simulink model "Leader"  (R2024b)
settings: Solver=ode4  StartTime=0  StopTime=100  FixedStep=0.001  RelTol=1e-3
undefined symbols (not defined in the file or in its folder): DiscIntNeverNeededParam
libraries: simulink x22, vrlib x1
(part 2 of 4)

== system Leader/Ardupilot Attitude Controller/Rate Controller/PID Pitch Rate/RAT_FLTT ==
  note: See AP_Math.cpp, calc_lowpass_alpha_dt()
  note: See AC_PID.cpp, update_all()
  note: Digital Filter:
      | $y_n = (1 - \alpha)y_{n-1} + x \cdot \alpha$
  note: Alpha Calculation: (Eqn is wrong, implementation is correct)
      | $\alpha = \frac{\mathrm{d}t}{\mathrm{d}t + 2 \pi T_{\mathrm{Cutoff}}$
  u : Inport
  cutoff_freq : Inport  Port=2
  ATC Sampling Time : Constant  Value=0.01
  Add : Sum
  Calculate Alpha : Product  Inputs=*/
  Compare To Zero : simulink/Logic and Bit Operations/Compare To Zero  relop=<=  OutDataTypeStr=boolean
  Compare To Zero1 : simulink/Logic and Bit Operations/Compare To Zero  relop=<=  OutDataTypeStr=boolean
  Constant2 : Constant
  Constant3 : Constant
  Constant4 : Constant
  Divide : Product  Inputs=*/
  Gain : Gain  Gain=2*pi
  Logical Operator : Logic  Operator=OR  AllPortsSameDT=off  OutDataTypeStr=boolean
  Product : Product
  Product1 : Product
  Subtract1 : Sum  Inputs=+-
  Sum : Sum  Inputs=++|  OutDataTypeStr=double
  Switch : Switch  Criteria=u2 > Threshold  SaturateOnIntegerOverflow=off  InputSameDT=off
  Unit Delay : UnitDelay  SampleTime=-1  HasFrameUpgradeWarning=on
  y : Outport
  wires:
  Constant4/1 -> Switch/1
  Logical Operator/1 -> Switch/2
  Compare To Zero1/1 -> Logical Operator/2
  Compare To Zero/1 -> Logical Operator/1
  [cutoff_freq] -> Compare To Zero1/1
  [dt] -> Compare To Zero/1
  Switch/1 -> [alpha]
  Product/1 -> Sum/1
  u/1 -> Product/2
  cutoff_freq/1 -> [cutoff_freq]
  [dt] -> Calculate Alpha/1, Add/1
  Add/1 -> Calculate Alpha/2
  Calculate Alpha/1 -> Switch/3
  [alpha] -> Product/1
  Constant2/1 -> Subtract1/1
  [alpha] -> Subtract1/2
  Subtract1/1 -> Product1/1
  Product1/1 -> Sum/2
  Unit Delay/1 -> Product1/2
  Sum/1 -> y/1, Unit Delay/1
  ATC Sampling Time/1 -> [dt]
  Constant3/1 -> Divide/1
  [cutoff_freq] -> Gain/1
  Gain/1 -> Divide/2
  Divide/1 -> Add/2

== system Leader/Ardupilot Attitude Controller/Rate Controller/PID Roll Rate/Calc Derivative ==
  e : Inport
  ATC Sampling Time : Constant  Value=0.01
  Divide : Product  Inputs=*/
  Sum : Sum  Inputs=|+-  OutDataTypeStr=double
  Unit Delay : UnitDelay  SampleTime=-1  HasFrameUpgradeWarning=on
  derivative : Outport
  wires:
  e/1 -> Sum/1, Unit Delay/1
  Unit Delay/1 -> Sum/2
  Sum/1 -> Divide/1
  Divide/1 -> derivative/1
  ATC Sampling Time/1 -> Divide/2

== system Leader/Ardupilot Attitude Controller/Rate Controller/PID Roll Rate/I ==
  note: Integrator, see AC_PID::update_i()
  e : Inport
  limitFlg : Inport  Port=2
  ki : Inport  Port=3
  i_max : Inport  Port=4
  ATC Sampling Time : Constant  Value=0.01
  Cast To Double : DataTypeConversion  OutDataTypeStr=double  SaturateOnIntegerOverflow=off  RndMeth=Floor
  Integrator : MATLAB Function  TreatAsAtomicUnit=on
  Unit Delay1 : UnitDelay  InitialCondition=0.0  SampleTime=-1  HasFrameUpgradeWarning=on
  integrator : Outport
  wires:
  [integrator_out] -> integrator/1
  ki/1 -> Integrator/4(ki)
  i_max/1 -> Integrator/5(i_max)
  e/1 -> Integrator/1(error)
  ATC Sampling Time/1 -> Integrator/6(dt)
  limitFlg/1 -> Integrator/3(limit_flg)
  [integrator_out] -> Unit Delay1/1
  Unit Delay1/1 -> Integrator/2(integrator)
  Integrator/1(integrator_out) -> Cast To Double/1
  Cast To Double/1 -> [integrator_out]

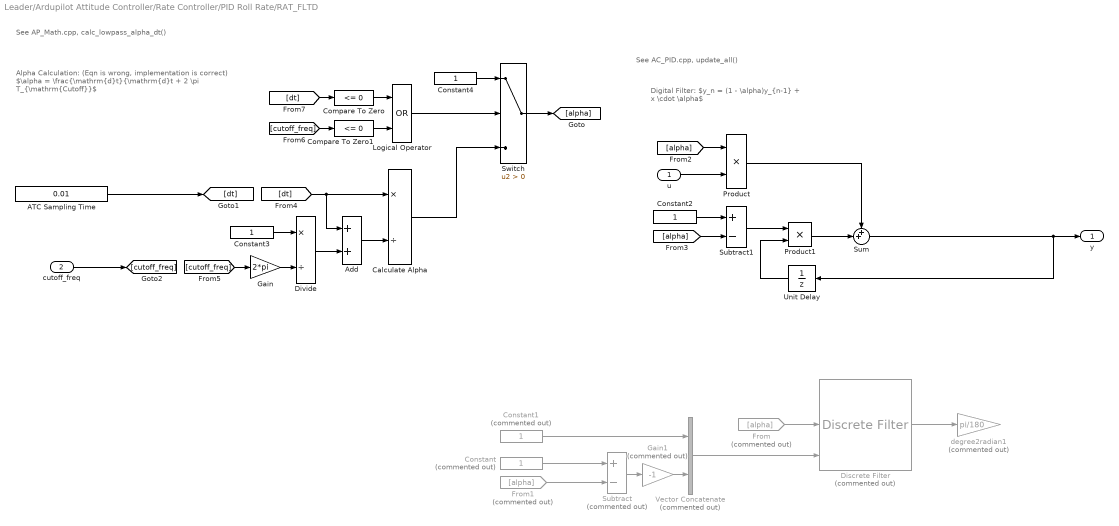
== system Leader/Ardupilot Attitude Controller/Rate Controller/PID Roll Rate/RAT_FLTD ==
  note: Digital Filter:
      | $y_n = (1 - \alpha)y_{n-1} + x \cdot \alpha$
  note: See AC_PID.cpp, update_all()
  note: See AP_Math.cpp, calc_lowpass_alpha_dt()
  note: Alpha Calculation: (Eqn is wrong, implementation is correct)
      | $\alpha = \frac{\mathrm{d}t}{\mathrm{d}t + 2 \pi T_{\mathrm{Cutoff}}$
  u : Inport
  cutoff_freq : Inport  Port=2
  ATC Sampling Time : Constant  Value=0.01
  Add : Sum
  Calculate Alpha : Product  Inputs=*/
  Compare To Zero : simulink/Logic and Bit Operations/Compare To Zero  relop=<=  OutDataTypeStr=boolean
  Compare To Zero1 : simulink/Logic and Bit Operations/Compare To Zero  relop=<=  OutDataTypeStr=boolean
  Constant : Constant  Commented=on
  Constant1 : Constant  Commented=on
  Constant2 : Constant
  Constant3 : Constant
  Constant4 : Constant
  Discrete Filter : DiscreteFilter  Commented=on  NumeratorSource=Input port  DenominatorSource=Input port  a0EqualsOne=on
      settings: InputPortMap=u0,p1,p3
  Divide : Product  Inputs=*/
  From : From  Commented=on  GotoTag=alpha
  From1 : From  Commented=on  GotoTag=alpha
  Gain : Gain  Gain=2*pi
  Gain1 : Gain  Commented=on  Gain=-1
  Logical Operator : Logic  Operator=OR  AllPortsSameDT=off  OutDataTypeStr=boolean
  Product : Product
  Product1 : Product
  Subtract : Sum  Commented=on  Inputs=+-
  Subtract1 : Sum  Inputs=+-
  Sum : Sum  Inputs=++|  OutDataTypeStr=double  AccumDataTypeStr=double
  Switch : Switch  Criteria=u2 > Threshold  SaturateOnIntegerOverflow=off  InputSameDT=off
  Unit Delay : UnitDelay  SampleTime=-1  HasFrameUpgradeWarning=on
  Vector Concatenate : Concatenate  Commented=on
  degree2radian1 : Gain  Commented=on  Gain=pi/180
  y : Outport
  wires:
  Product1/1 -> Sum/2
  Unit Delay/1 -> Product1/2
  Subtract1/1 -> Product1/1
  [alpha] -> Subtract1/2
  Constant2/1 -> Subtract1/1
  [alpha] -> Product/1
  Vector Concatenate/1 -> Discrete Filter/3
  Constant1/1 -> Vector Concatenate/1
  Gain1/1 -> Vector Concatenate/2
  Subtract/1 -> Gain1/1
  Constant/1 -> Subtract/1
  From1/1 -> Subtract/2
  From/1 -> Discrete Filter/2
  Calculate Alpha/1 -> Switch/3
  Add/1 -> Calculate Alpha/2
  [dt] -> Add/1, Calculate Alpha/1
  Gain/1 -> Divide/2
  cutoff_freq/1 -> [cutoff_freq]
  Discrete Filter/1 -> degree2radian1/1
  u/1 -> Product/2
  Divide/1 -> Add/2
  Constant3/1 -> Divide/1
  Product/1 -> Sum/1
  Switch/1 -> [alpha]
  [cutoff_freq] -> Gain/1
  [dt] -> Compare To Zero/1
  [cutoff_freq] -> Compare To Zero1/1
  Compare To Zero/1 -> Logical Operator/1
  Compare To Zero1/1 -> Logical Operator/2
  Logical Operator/1 -> Switch/2
  Constant4/1 -> Switch/1
  Sum/1 -> Unit Delay/1, y/1
  ATC Sampling Time/1 -> [dt]

== system Leader/Ardupilot Attitude Controller/Rate Controller/PID Roll Rate/RAT_FLTE ==
  note: Digital Filter:
      | $y_n = (1 - \alpha)y_{n-1} + x \cdot \alpha$
  note: See AC_PID.cpp, update_all()
  note: See AP_Math.cpp, calc_lowpass_alpha_dt()
  note: Alpha Calculation: (Eqn is wrong, implementation is correct)
      | $\alpha = \frac{\mathrm{d}t}{\mathrm{d}t + 2 \pi T_{\mathrm{Cutoff}}$
  u : Inport
  cutoff_freq : Inport  Port=2
  ATC Sampling Time : Constant  Value=0.01
  Add : Sum
  Calculate Alpha : Product  Inputs=*/
  Compare To Zero : simulink/Logic and Bit Operations/Compare To Zero  relop=<=  OutDataTypeStr=boolean
  Compare To Zero1 : simulink/Logic and Bit Operations/Compare To Zero  relop=<=  OutDataTypeStr=boolean
  Constant2 : Constant
  Constant3 : Constant
  Constant4 : Constant
  Divide : Product  Inputs=*/
  Gain : Gain  Gain=2*pi
  Logical Operator : Logic  Operator=OR  AllPortsSameDT=off  OutDataTypeStr=boolean
  Product : Product
  Product1 : Product
  Subtract1 : Sum  Inputs=+-
  Sum : Sum  Inputs=++|  OutDataTypeStr=double
  Switch : Switch  Criteria=u2 > Threshold  SaturateOnIntegerOverflow=off  InputSameDT=off
  Unit Delay : UnitDelay  SampleTime=-1  HasFrameUpgradeWarning=on
  y : Outport
  wires:
  Product1/1 -> Sum/2
  Unit Delay/1 -> Product1/2
  Subtract1/1 -> Product1/1
  [alpha] -> Subtract1/2
  Constant2/1 -> Subtract1/1
  [alpha] -> Product/1
  Calculate Alpha/1 -> Switch/3
  Add/1 -> Calculate Alpha/2
  [dt] -> Add/1, Calculate Alpha/1
  cutoff_freq/1 -> [cutoff_freq]
  u/1 -> Product/2
  Product/1 -> Sum/1
  Switch/1 -> [alpha]
  [dt] -> Compare To Zero/1
  [cutoff_freq] -> Compare To Zero1/1
  Compare To Zero/1 -> Logical Operator/1
  Compare To Zero1/1 -> Logical Operator/2
  Logical Operator/1 -> Switch/2
  Constant4/1 -> Switch/1
  Sum/1 -> Unit Delay/1, y/1
  ATC Sampling Time/1 -> [dt]
  [cutoff_freq] -> Gain/1
  Divide/1 -> Add/2
  Constant3/1 -> Divide/1
  Gain/1 -> Divide/2

== system Leader/Ardupilot Attitude Controller/Rate Controller/PID Roll Rate/RAT_FLTT ==
  note: See AP_Math.cpp, calc_lowpass_alpha_dt()
  note: See AC_PID.cpp, update_all()
  note: Digital Filter:
      | $y_n = (1 - \alpha)y_{n-1} + x \cdot \alpha$
  note: Alpha Calculation: (Eqn is wrong, implementation is correct)
      | $\alpha = \frac{\mathrm{d}t}{\mathrm{d}t + 2 \pi T_{\mathrm{Cutoff}}$
  u : Inport
  cutoff_freq : Inport  Port=2
  ATC Sampling Time : Constant  Value=0.01
  Add : Sum
  Calculate Alpha : Product  Inputs=*/
  Compare To Zero : simulink/Logic and Bit Operations/Compare To Zero  relop=<=  OutDataTypeStr=boolean
  Compare To Zero1 : simulink/Logic and Bit Operations/Compare To Zero  relop=<=  OutDataTypeStr=boolean
  Constant2 : Constant
  Constant3 : Constant
  Constant4 : Constant
  Divide : Product  Inputs=*/
  Gain : Gain  Gain=2*pi
  Logical Operator : Logic  Operator=OR  AllPortsSameDT=off  OutDataTypeStr=boolean
  Product : Product
  Product1 : Product
  Subtract1 : Sum  Inputs=+-
  Sum : Sum  Inputs=++|  OutDataTypeStr=double
  Switch : Switch  Criteria=u2 > Threshold  SaturateOnIntegerOverflow=off  InputSameDT=off
  Unit Delay : UnitDelay  SampleTime=-1  HasFrameUpgradeWarning=on
  y : Outport
  wires:
  Constant4/1 -> Switch/1
  Logical Operator/1 -> Switch/2
  Compare To Zero1/1 -> Logical Operator/2
  Compare To Zero/1 -> Logical Operator/1
  [cutoff_freq] -> Compare To Zero1/1
  [dt] -> Compare To Zero/1
  Switch/1 -> [alpha]
  Product/1 -> Sum/1
  u/1 -> Product/2
  cutoff_freq/1 -> [cutoff_freq]
  [dt] -> Calculate Alpha/1, Add/1
  Add/1 -> Calculate Alpha/2
  Calculate Alpha/1 -> Switch/3
  [alpha] -> Product/1
  Constant2/1 -> Subtract1/1
  [alpha] -> Subtract1/2
  Subtract1/1 -> Product1/1
  Product1/1 -> Sum/2
  Unit Delay/1 -> Product1/2
  Sum/1 -> y/1, Unit Delay/1
  ATC Sampling Time/1 -> [dt]
  Constant3/1 -> Divide/1
  [cutoff_freq] -> Gain/1
  Gain/1 -> Divide/2
  Divide/1 -> Add/2

== system Leader/Ardupilot Attitude Controller/Rate Controller/PID Yaw Rate/Calc Derivative ==
  e : Inport
  ATC Sampling Time : Constant  Value=0.01
  Divide : Product  Inputs=*/
  Sum : Sum  Inputs=|+-  OutDataTypeStr=double
  Unit Delay : UnitDelay  SampleTime=-1  HasFrameUpgradeWarning=on
  derivative : Outport
  wires:
  e/1 -> Sum/1, Unit Delay/1
  Unit Delay/1 -> Sum/2
  Sum/1 -> Divide/1
  Divide/1 -> derivative/1
  ATC Sampling Time/1 -> Divide/2

== system Leader/Ardupilot Attitude Controller/Rate Controller/PID Yaw Rate/I ==
  note: Integrator, see AC_PID::update_i()
  e : Inport
  limitFlg : Inport  Port=2
  ki : Inport  Port=3
  i_max : Inport  Port=4
  ATC Sampling Time : Constant  Value=0.01
  Integrator : MATLAB Function  TreatAsAtomicUnit=on
  Unit Delay1 : UnitDelay  SampleTime=-1  HasFrameUpgradeWarning=on
  integrator : Outport
  wires:
  [integrator_out] -> integrator/1
  [integrator_out] -> Unit Delay1/1
  Integrator/1(integrator_out) -> [integrator_out]
  Unit Delay1/1 -> Integrator/2(integrator)
  ki/1 -> Integrator/4(ki)
  i_max/1 -> Integrator/5(i_max)
  e/1 -> Integrator/1(error)
  ATC Sampling Time/1 -> Integrator/6(dt)
  limitFlg/1 -> Integrator/3(limit_flg)

== system Leader/Ardupilot Attitude Controller/Rate Controller/PID Yaw Rate/RAT_FLTD ==
  note: Digital Filter:
      | $y_n = (1 - \alpha)y_{n-1} + x \cdot \alpha$
  note: See AC_PID.cpp, update_all()
  note: See AP_Math.cpp, calc_lowpass_alpha_dt()
  note: Alpha Calculation: (Eqn is wrong, implementation is correct)
      | $\alpha = \frac{\mathrm{d}t}{\mathrm{d}t + 2 \pi T_{\mathrm{Cutoff}}$
  u : Inport
  cutoff_freq : Inport  Port=2
  ATC Sampling Time : Constant  Value=0.01
  Add : Sum
  Calculate Alpha : Product  Inputs=*/
  Compare To Zero : simulink/Logic and Bit Operations/Compare To Zero  relop=<=  OutDataTypeStr=boolean
  Compare To Zero1 : simulink/Logic and Bit Operations/Compare To Zero  relop=<=  OutDataTypeStr=boolean
  Constant2 : Constant
  Constant3 : Constant
  Constant4 : Constant
  Divide : Product  Inputs=*/
  Gain : Gain  Gain=2*pi
  Logical Operator : Logic  Operator=OR  AllPortsSameDT=off  OutDataTypeStr=boolean
  Product : Product
  Product1 : Product
  Subtract1 : Sum  Inputs=+-
  Sum : Sum  Inputs=++|  OutDataTypeStr=double
  Switch : Switch  Criteria=u2 > Threshold  SaturateOnIntegerOverflow=off  InputSameDT=off
  Unit Delay : UnitDelay  SampleTime=-1  HasFrameUpgradeWarning=on
  y : Outport
  wires:
  Product1/1 -> Sum/2
  Unit Delay/1 -> Product1/2
  Subtract1/1 -> Product1/1
  [alpha] -> Subtract1/2
  Constant2/1 -> Subtract1/1
  [alpha] -> Product/1
  Calculate Alpha/1 -> Switch/3
  Add/1 -> Calculate Alpha/2
  [dt] -> Add/1, Calculate Alpha/1
  Gain/1 -> Divide/2
  cutoff_freq/1 -> [cutoff_freq]
  u/1 -> Product/2
  Divide/1 -> Add/2
  Constant3/1 -> Divide/1
  Product/1 -> Sum/1
  Switch/1 -> [alpha]
  [cutoff_freq] -> Gain/1
  [dt] -> Compare To Zero/1
  [cutoff_freq] -> Compare To Zero1/1
  Compare To Zero/1 -> Logical Operator/1
  Compare To Zero1/1 -> Logical Operator/2
  Logical Operator/1 -> Switch/2
  Constant4/1 -> Switch/1
  Sum/1 -> Unit Delay/1, y/1
  ATC Sampling Time/1 -> [dt]

== system Leader/Ardupilot Attitude Controller/Rate Controller/PID Yaw Rate/RAT_FLTE ==
  note: Digital Filter:
      | $y_n = (1 - \alpha)y_{n-1} + x \cdot \alpha$
  note: See AC_PID.cpp, update_all()
  note: See AP_Math.cpp, calc_lowpass_alpha_dt()
  note: Alpha Calculation: (Eqn is wrong, implementation is correct)
      | $\alpha = \frac{\mathrm{d}t}{\mathrm{d}t + 2 \pi T_{\mathrm{Cutoff}}$
  u : Inport
  cutoff_freq : Inport  Port=2
  ATC Sampling Time : Constant  Value=0.01
  Add : Sum
  Calculate Alpha : Product  Inputs=*/
  Compare To Zero : simulink/Logic and Bit Operations/Compare To Zero  relop=<=  OutDataTypeStr=boolean
  Compare To Zero1 : simulink/Logic and Bit Operations/Compare To Zero  relop=<=  OutDataTypeStr=boolean
  Constant2 : Constant
  Constant3 : Constant
  Constant4 : Constant
  Divide : Product  Inputs=*/
  Gain : Gain  Gain=2*pi
  Logical Operator : Logic  Operator=OR  AllPortsSameDT=off  OutDataTypeStr=boolean
  Product : Product
  Product1 : Product
  Subtract1 : Sum  Inputs=+-
  Sum : Sum  Inputs=++|  OutDataTypeStr=double
  Switch : Switch  Criteria=u2 > Threshold  SaturateOnIntegerOverflow=off  InputSameDT=off
  Unit Delay : UnitDelay  SampleTime=-1  HasFrameUpgradeWarning=on
  y : Outport
  wires:
  Product1/1 -> Sum/2
  Unit Delay/1 -> Product1/2
  Subtract1/1 -> Product1/1
  [alpha] -> Subtract1/2
  Constant2/1 -> Subtract1/1
  [alpha] -> Product/1
  Calculate Alpha/1 -> Switch/3
  Add/1 -> Calculate Alpha/2
  [dt] -> Add/1, Calculate Alpha/1
  cutoff_freq/1 -> [cutoff_freq]
  u/1 -> Product/2
  Product/1 -> Sum/1
  Switch/1 -> [alpha]
  [dt] -> Compare To Zero/1
  [cutoff_freq] -> Compare To Zero1/1
  Compare To Zero/1 -> Logical Operator/1
  Compare To Zero1/1 -> Logical Operator/2
  Logical Operator/1 -> Switch/2
  Constant4/1 -> Switch/1
  Sum/1 -> Unit Delay/1, y/1
  ATC Sampling Time/1 -> [dt]
  [cutoff_freq] -> Gain/1
  Divide/1 -> Add/2
  Constant3/1 -> Divide/1
  Gain/1 -> Divide/2

== system Leader/Ardupilot Attitude Controller/Rate Controller/PID Yaw Rate/RAT_FLTT ==
  note: See AP_Math.cpp, calc_lowpass_alpha_dt()
  note: See AC_PID.cpp, update_all()
  note: Digital Filter:
      | $y_n = (1 - \alpha)y_{n-1} + x \cdot \alpha$
  note: Alpha Calculation: (Eqn is wrong, implementation is correct)
      | $\alpha = \frac{\mathrm{d}t}{\mathrm{d}t + 2 \pi T_{\mathrm{Cutoff}}$
  u : Inport
  cutoff_freq : Inport  Port=2
  ATC Sampling Time : Constant  Value=0.01
  Add : Sum
  Calculate Alpha : Product  Inputs=*/
  Compare To Zero : simulink/Logic and Bit Operations/Compare To Zero  relop=<=  OutDataTypeStr=boolean
  Compare To Zero1 : simulink/Logic and Bit Operations/Compare To Zero  relop=<=  OutDataTypeStr=boolean
  Constant2 : Constant
  Constant3 : Constant
  Constant4 : Constant
  Divide : Product  Inputs=*/
  Gain : Gain  Gain=2*pi
  Logical Operator : Logic  Operator=OR  AllPortsSameDT=off  OutDataTypeStr=boolean
  Product : Product
  Product1 : Product
  Subtract1 : Sum  Inputs=+-
  Sum : Sum  Inputs=++|  OutDataTypeStr=double
  Switch : Switch  Criteria=u2 > Threshold  SaturateOnIntegerOverflow=off  InputSameDT=off
  Unit Delay : UnitDelay  SampleTime=-1  HasFrameUpgradeWarning=on
  y : Outport
  wires:
  Constant4/1 -> Switch/1
  Logical Operator/1 -> Switch/2
  Compare To Zero1/1 -> Logical Operator/2
  Compare To Zero/1 -> Logical Operator/1
  [cutoff_freq] -> Compare To Zero1/1
  [dt] -> Compare To Zero/1
  Switch/1 -> [alpha]
  Product/1 -> Sum/1
  u/1 -> Product/2
  cutoff_freq/1 -> [cutoff_freq]
  [dt] -> Calculate Alpha/1, Add/1
  Add/1 -> Calculate Alpha/2
  Calculate Alpha/1 -> Switch/3
  [alpha] -> Product/1
  Constant2/1 -> Subtract1/1
  [alpha] -> Subtract1/2
  Subtract1/1 -> Product1/1
  Product1/1 -> Sum/2
  Unit Delay/1 -> Product1/2
  Sum/1 -> y/1, Unit Delay/1
  ATC Sampling Time/1 -> [dt]
  Constant3/1 -> Divide/1
  [cutoff_freq] -> Gain/1
  Gain/1 -> Divide/2
  Divide/1 -> Add/2

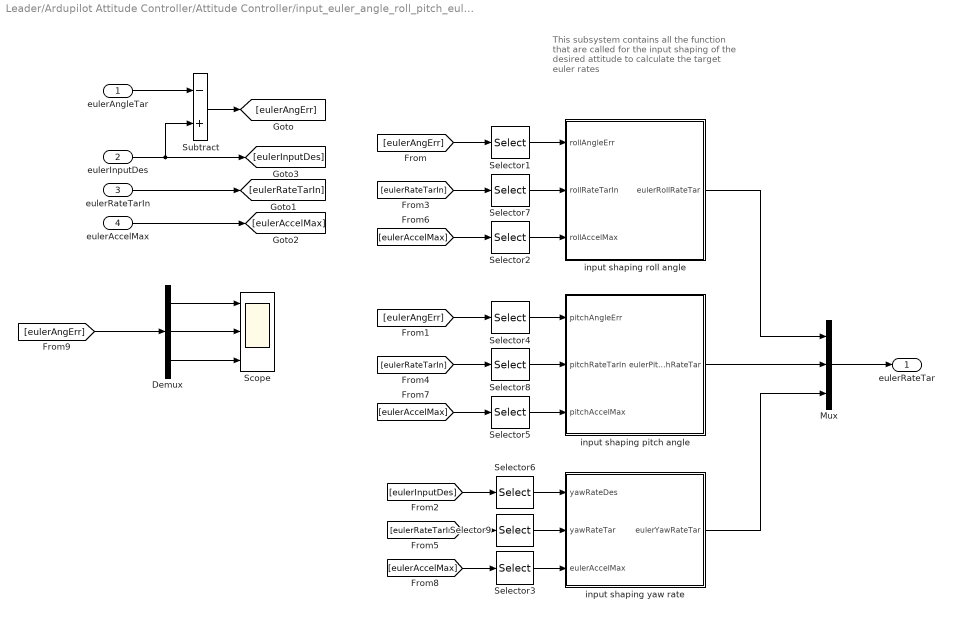
== system Leader/Ardupilot Attitude Controller/Attitude Controller/input_euler_angle_roll_pitch_euler_rate_yaw()/Feedforward enabled/input shaping ==
  note: This subsystem contains all the function that are called for the input shaping of the desired attitude to calculate the target euler rates
  eulerAngleTar : Inport
  eulerInputDes : Inport  Port=2
  eulerRateTarIn : Inport  Port=3
  eulerAccelMax : Inport  Port=4
  Demux : Demux  Outputs=3
  Mux : Mux  Inputs=3
  Scope : Scope  NumInputPorts=3
  Selector1 : Selector  InputPortWidth=3  IndexOptions=Index vector (dialog)  Indices=[1]  OutputSizes=1
  Selector2 : Selector  InputPortWidth=3  IndexOptions=Index vector (dialog)  Indices=[1]  OutputSizes=1
  Selector3 : Selector  InputPortWidth=3  IndexOptions=Index vector (dialog)  Indices=[3]  OutputSizes=1
  Selector4 : Selector  InputPortWidth=3  IndexOptions=Index vector (dialog)  Indices=[2]  OutputSizes=1
  Selector5 : Selector  InputPortWidth=3  IndexOptions=Index vector (dialog)  Indices=[2]  OutputSizes=1
  Selector6 : Selector  InputPortWidth=3  IndexOptions=Index vector (dialog)  Indices=[3]  OutputSizes=1
  Selector7 : Selector  InputPortWidth=3  IndexOptions=Index vector (dialog)  Indices=[1]  OutputSizes=1
  Selector8 : Selector  InputPortWidth=3  IndexOptions=Index vector (dialog)  Indices=[2]  OutputSizes=1
  Selector9 : Selector  InputPortWidth=3  IndexOptions=Index vector (dialog)  Indices=[3]  OutputSizes=1
  Subtract : Sum  Inputs=-+
  input shaping pitch angle : Subsystem
  input shaping roll angle : Subsystem
  input shaping yaw rate : Subsystem
  eulerRateTar : Outport
  wires:
  eulerAngleTar/1 -> Subtract/1
  eulerInputDes/1 -> [eulerInputDes], Subtract/2
  Selector1/1 -> input shaping roll angle/1(rollAngleErr)
  Selector2/1 -> input shaping roll angle/3(rollAccelMax)
  Selector3/1 -> input shaping yaw rate/3(eulerAccelMax)
  Selector6/1 -> input shaping yaw rate/1(yawRateDes)
  Selector7/1 -> input shaping roll angle/2(rollRateTarIn)
  Selector4/1 -> input shaping pitch angle/1(pitchAngleErr)
  Selector5/1 -> input shaping pitch angle/3(pitchAccelMax)
  Selector8/1 -> input shaping pitch angle/2(pitchRateTarIn)
  Selector9/1 -> input shaping yaw rate/2(yawRateTar)
  Mux/1 -> eulerRateTar/1
  input shaping roll angle/1(eulerRollRateTar) -> Mux/1
  input shaping pitch angle/1(eulerPitchRateTar) -> Mux/2
  input shaping yaw rate/1(eulerYawRateTar) -> Mux/3
  Subtract/1 -> [eulerAngErr]
  eulerRateTarIn/1 -> [eulerRateTarIn]
  eulerAccelMax/1 -> [eulerAccelMax]
  [eulerAngErr] -> Selector1/1
  [eulerAngErr] -> Selector4/1
  [eulerInputDes] -> Selector6/1
  [eulerRateTarIn] -> Selector7/1
  [eulerRateTarIn] -> Selector8/1
  [eulerRateTarIn] -> Selector9/1
  [eulerAccelMax] -> Selector2/1
  [eulerAccelMax] -> Selector5/1
  [eulerAccelMax] -> Selector3/1
  Demux/2 -> Scope/2
  [eulerAngErr] -> Demux/1
  Demux/1 -> Scope/1
  Demux/3 -> Scope/3

== system Leader/Ardupilot Attitude Controller/Attitude Controller/input_euler_angle_roll_pitch_euler_rate_yaw()/Update attitudeTarget/Rotate target attitude ==
  attitudeTarget : Inport
  angVelTar : Inport  Port=2
  MATLAB Function1 : MATLAB Function  TreatAsAtomicUnit=on
  MATLAB Function5 : MATLAB Function  TreatAsAtomicUnit=on
  Product : Product
  dt : Constant  Value=0.01
  attitudeTargetRot : Outport
  wires:
  Product/1 -> MATLAB Function5/1(vec)
  angVelTar/1 -> Product/1
  dt/1 -> Product/2
  MATLAB Function5/1(q) -> MATLAB Function1/2(q2)  "attitudeTargetUpdate"
  attitudeTarget/1 -> MATLAB Function1/1(q1)
  MATLAB Function1/1(qRes) -> attitudeTargetRot/1  "attitudeTargetRot"

== system Leader/Ardupilot Attitude Controller/Attitude Controller/input_euler_angle_roll_pitch_euler_rate_yaw()/thrust_heading_rotation_angles()/Yaw error limitation ==
  note: Output adapted attitudeTarget and attitudeError if yaw limiting condition is met. Otherwise output old values.
  note: Limiting condition: if(!iszero(_p_angle_yaw.kp()) && abs(attitude_error.z) > ACCEL_Y_CONTROLLER_MAX_RADSS / _p_angle_yaw.kp())
      | --> P gain of yaw angle controller is not zero AND yaw attitude error is greater than max. yaw acceleration divided by p gain
  note: Limiting of the yaw error based on the maximum allowed yaw acceleration.
      | attitudeError and attitudeTarget are updated to include the applied limits.
  attitudeErrorIn : Inport
  thrustVecCorrection : Inport  Port=2
  attitudeBody : Inport  Port=3
  attitudeTarget : Inport  Port=4
  AND : Logic  AllPortsSameDT=off  OutDataTypeStr=boolean
  ATC.ACCEL_Y_CONTROLLER_MAX_RADSS : Constant  Value=2.0944
  ATC.ANG_YAW_P : Constant  Value=8.0
  Abs : Abs  SaturateOnIntegerOverflow=off
  Divide : Product  Inputs=*/
  GreaterThan : RelationalOperator  Operator=>  OutDataTypeStr=boolean  RndMeth=Simplest  InputSameDT=off
  IsNonZero : simulink/Logic and Bit Operations/Compare To Zero  relop=~=  OutDataTypeStr=boolean
  Selector : Selector  InputPortWidth=3  IndexOptions=Index vector (dialog)  Indices=[3]  OutputSizes=1
  Switch : Switch  Criteria=u2 > Threshold  SaturateOnIntegerOverflow=off  InputSameDT=off
  Switch1 : Switch  Criteria=u2 > Threshold  SaturateOnIntegerOverflow=off  InputSameDT=off
  Yaw limiting and recalculation of attitudeTarget : Subsystem
  atitudeTarget : Outport
  attitudeError : Outport  Port=2
  wires:
  [attitudeError] -> Selector/1
  Divide/1 -> GreaterThan/2
  Selector/1 -> Abs/1
  Abs/1 -> GreaterThan/1
  GreaterThan/1 -> AND/1
  ATC.ANG_YAW_P/1 -> IsNonZero/1, Divide/2
  IsNonZero/1 -> AND/2
  attitudeErrorIn/1 -> [attitudeError]
  AND/1 -> Yaw limiting and recalculation of attitudeTarget/Enable, Switch1/2, Switch/2
  [attitudeError] -> Yaw limiting and recalculation of attitudeTarget/1(attitudeErrorIn)
  thrustVecCorrection/1 -> Yaw limiting and recalculation of attitudeTarget/2(thrustVecCorrection)
  attitudeBody/1 -> Yaw limiting and recalculation of attitudeTarget/3(attitudeBody)
  Yaw limiting and recalculation of attitudeTarget/1(attitudeTarget) -> Switch/1
  Yaw limiting and recalculation of attitudeTarget/2(attitudeError) -> Switch1/1
  attitudeTarget/1 -> Switch/3
  [attitudeError] -> Switch1/3
  Switch/1 -> atitudeTarget/1
  Switch1/1 -> attitudeError/1
  ATC.ACCEL_Y_CONTROLLER_MAX_RADSS/1 -> Divide/1

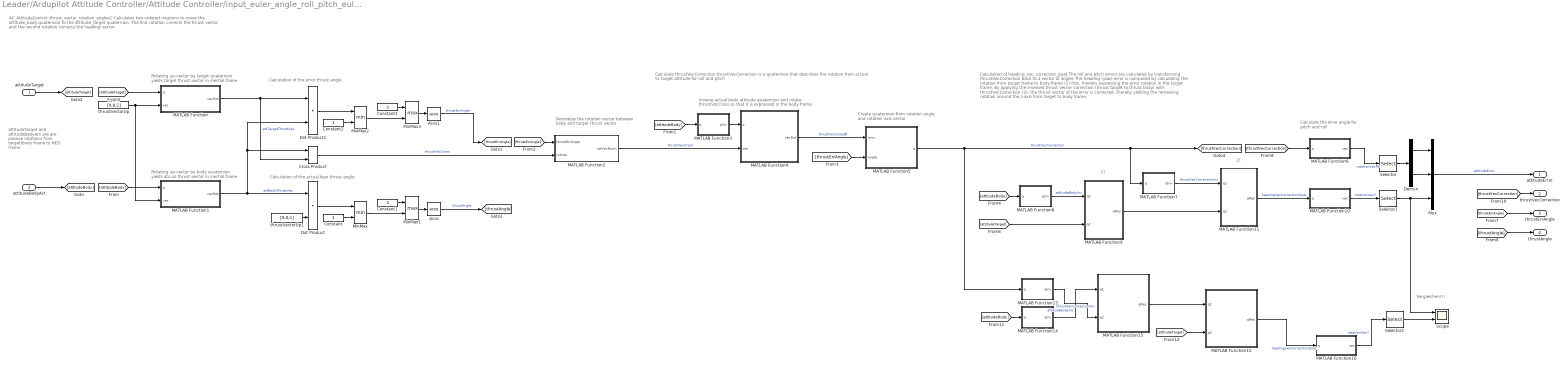
== system Leader/Ardupilot Attitude Controller/Attitude Controller/input_euler_angle_roll_pitch_euler_rate_yaw()/thrust_heading_rotation_angles()/thrust_vector_rotation_angles() ==
  note: Vergleichen!!!
  note: 1)
  note: attitudeTarget and
      | attitudeBodyAct are are passive rotations from target/body frame to NED frame
  note: Calculation of heading_vec_correction_quat
      | The roll and pitch errors are calculated by transforming thrustVecCorrection back to a vector of angles
      | The heading (yaw) error is computed by calculating the rotation from target frame to body-frame (1) first, thereby expressing the error rotation in the target frame. By applying the inversed thrust vector correction (thrust target to thrust body) with thrustVecCorrection (2), the thrust vector of the error is corrected, thereby yielding the remaining rotation around the z-axis from target to body frame.
  note: Create quaternion from rotation angle and rotation axis vector
  note: Inverse actual body attitude quaternion and rotate thrustVecCross so that it is expressed in the body frame.
  note: Calculate the error angle for pitch and roll
  note: Calculate thrustVecCorrection
      | thrustVecCorrection is a quaternion that describes the rotation from actual to target attitude for roll and pitch
  note: Normalize the rotation vector between body and target thrust vector
  note: Calculation of the actual lean thrust angle
  note: Rotating up-vector by target quaternion
      | yields target thrust vector in inertial frame
  note: AC_AttitudeControl::thrust_vector_rotation_angles()
      | Calculates two ordered rotations to move the attitude_body quaternion to the attitude_target quaternion. The first rotation corrects the thrust vector and the second rotation corrects the heading vector.
  note: Rotating up-vector by body quaternion
      | yields atcual thrust vector in inertial frame
  note: Calculation of the error thrust angle
  note: 2)
  attitudeTarget : Inport
  attitudeBodyAct : Inport  Port=2
  Acos : Trigonometry  Operator=acos
  Acos1 : Trigonometry  Operator=acos
  Constant : Constant
  Constant1 : Constant  Value=-1
  Constant2 : Constant
  Constant3 : Constant  Value=-1
  Cross Product : vrlib/Utilities/Cross Product
  Demux : Demux  Outputs=2
  Dot Product : DotProduct  OutDataTypeStr=Inherit: Inherit via internal rule
  Dot Product1 : DotProduct  OutDataTypeStr=Inherit: Inherit via internal rule
  MATLAB Function : MATLAB Function  TreatAsAtomicUnit=on
  MATLAB Function1 : MATLAB Function  TreatAsAtomicUnit=on
  MATLAB Function10 : MATLAB Function  TreatAsAtomicUnit=on
  MATLAB Function11 : MATLAB Function  TreatAsAtomicUnit=on
  MATLAB Function12 : MATLAB Function  TreatAsAtomicUnit=on
  MATLAB Function13 : MATLAB Function  TreatAsAtomicUnit=on
  MATLAB Function14 : MATLAB Function  TreatAsAtomicUnit=on
  MATLAB Function15 : MATLAB Function  TreatAsAtomicUnit=on
  MATLAB Function16 : MATLAB Function  TreatAsAtomicUnit=on
  MATLAB Function2 : MATLAB Function  TreatAsAtomicUnit=on
  MATLAB Function3 : MATLAB Function  TreatAsAtomicUnit=on
  MATLAB Function4 : MATLAB Function  TreatAsAtomicUnit=on
  MATLAB Function5 : MATLAB Function  TreatAsAtomicUnit=on
  MATLAB Function6 : MATLAB Function  TreatAsAtomicUnit=on
  MATLAB Function7 : MATLAB Function  TreatAsAtomicUnit=on
  MATLAB Function8 : MATLAB Function  TreatAsAtomicUnit=on
  MATLAB Function9 : MATLAB Function  TreatAsAtomicUnit=on
  MinMax : MinMax  Inputs=2
  MinMax1 : MinMax  Function=max  Inputs=2
  MinMax2 : MinMax  Inputs=2
  MinMax3 : MinMax  Function=max  Inputs=2
  Mux : Mux  Inputs=3
  Scope : Scope  NumInputPorts=2
  Selector : Selector  InputPortWidth=3  IndexOptions=Index vector (dialog)  Indices=[1 2]  OutputSizes=1
  Selector1 : Selector  InputPortWidth=3  IndexOptions=Index vector (dialog)  Indices=[3]  OutputSizes=1
  Selector2 : Selector  InputPortWidth=3  IndexOptions=Index vector (dialog)  Indices=[3]  OutputSizes=1
  thrustVectorUp : Constant  Value=[0;0;1]  OutDataTypeStr=double
  thrustVectorUp1 : Constant  Value=[0;0;1]  OutDataTypeStr=double
  attitudeError : Outport
  thrustVecCorrection : Outport  Port=2
  thrustErrAngle : Outport  Port=3
  thrustAngle : Outport  Port=4
  wires:
  attitudeTarget/1 -> [attitudeTarget]
  thrustVectorUp/1 -> MATLAB Function1/2(vec), MATLAB Function/2(vec)
  [attitudeBody] -> MATLAB Function1/1(q)
  MATLAB Function/1(vecRot) -> Cross Product/2, Dot Product1/1  "attTargetThrustVec"
  MATLAB Function1/1(vecRot) -> Dot Product/1, Cross Product/1, Dot Product1/2  "attBodyThrustVec"
  Dot Product/1 -> MinMax/1
  MinMax/1 -> MinMax1/2
  Constant/1 -> MinMax/2
  Constant1/1 -> MinMax1/1
  MinMax1/1 -> Acos/1
  thrustVectorUp1/1 -> Dot Product/2
  Acos/1 -> [thrustAngle]  "thrustAngle"
  Constant2/1 -> MinMax2/2
  Dot Product1/1 -> MinMax2/1
  Constant3/1 -> MinMax3/1
  MinMax3/1 -> Acos1/1
  MinMax2/1 -> MinMax3/2
  Acos1/1 -> [thrustErrAngle]  "thrustErrAngle"
  attitudeBodyAct/1 -> [attitudeBody]
  [attitudeBody] -> MATLAB Function3/1(q)
  MATLAB Function2/1(rotVecNorm) -> MATLAB Function4/2(vec)  "thrustVecCross"
  MATLAB Function3/1(qInv) -> MATLAB Function4/1(q)
  [thrustErrAngle] -> MATLAB Function2/1(thrustErrAngle)
  MATLAB Function4/1(vecRot) -> MATLAB Function5/1(axis)  "thrustVecCrossBf"
  [thrustErrAngle] -> MATLAB Function5/2(angle)
  [attitudeBody] -> MATLAB Function8/1(q)
  [attitudeTarget] -> MATLAB Function/1(q)
  MATLAB Function7/1(qInv) -> MATLAB Function11/1(q1)  "thrustVecCorrectionInv"
  MATLAB Function8/1(qInv) -> MATLAB Function9/1(q1)  "attitudeBodyInv"
  [attitudeTarget] -> MATLAB Function9/2(q2)
  MATLAB Function11/1(qRes) -> MATLAB Function10/1(q)  "headingVecCorrectionQuat"
  MATLAB Function10/1(vec) -> Selector1/1  "rotationVecY"
  MATLAB Function6/1(vec) -> Selector/1  "rotationVecRP"
  Demux/1 -> Mux/1
  Demux/2 -> Mux/2
  Selector/1 -> Demux/1
  Selector1/1 -> Scope/1, Mux/3
  Mux/1 -> attitudeError/1  "attitudeError"
  [thrustErrAngle] -> thrustErrAngle/1
  [thrustAngle] -> thrustAngle/1
  [thrustVecCorrection] -> MATLAB Function6/1(q)
  [thrustVecCorrection] -> thrustVecCorrection/1
  [attitudeTarget] -> MATLAB Function12/2(q2)
  MATLAB Function15/1(qRes) -> MATLAB Function12/1(q1)
  MATLAB Function14/1(qInv) -> MATLAB Function15/1(q1)  "attitudeBodyInv"
  MATLAB Function13/1(qInv) -> MATLAB Function15/2(q2)  "thrustVecCorrectionInv"
  [attitudeBody] -> MATLAB Function14/1(q)
  MATLAB Function5/1(q) -> MATLAB Function13/1(q), [thrustVecCorrection], MATLAB Function7/1(q)  "thrustVecCorrection"
  MATLAB Function9/1(qRes) -> MATLAB Function11/2(q2)
  MATLAB Function12/1(qRes) -> MATLAB Function16/1(q)  "headingVecCorrectionQuat"
  MATLAB Function16/1(vec) -> Selector2/1  "rotationVecY"
  Selector2/1 -> Scope/2
  Cross Product/1 -> MATLAB Function2/2(rotVec)  "thrustVecCross"

== system Leader/Ardupilot Attitude Controller/Attitude Controller/input_euler_angle_roll_pitch_euler_rate_yaw()/update_ang_vel_target_from_att_error()/Calc angular velocity target pitch ==
  note: Use square root controller if maximum angular acceleration is not zero
  attitudeErrorPitch : Inport
  ATC.ACCEL_P_MAX : Constant  Commented=on  Value=108000
  ATC.ACCEL_P_MAX - 1 : Constant  Commented=on  Value=108000
  ATC.ACCEL_RP_CONTROLLER_MAX_RADSS : Constant  Value=720
  ATC.ACCEL_RP_CONTROLLER_MIN_RADSS : Constant  Value=40
  ATC.ANG_PIT_P : Constant  Value=4.5
  ATC.ANG_PIT_P - 1 : Constant  Value=6.0
  Constant : Constant  Value=0
  Constant1 : Constant  Value=0
  Gain1 : Gain  Gain=0.5
  Product : Product
  Saturation Dynamic : simulink/Discontinuities/Saturation Dynamic  OutMin=[]  OutMax=[]  OutDataTypeStr=Inherit: Same as second input  OutDataType=fixdt(1, 16)  OutScaling=2^-10  DoSatur=off
  Square Root Controller : MATLAB Function  TreatAsAtomicUnit=on
  Switch : Switch  Criteria=u2 > Threshold  SaturateOnIntegerOverflow=off  InputSameDT=off
  cdeg/ss to rad/ss : Gain  Gain=0.01*pi/180
  cdeg/ss to rad/ss - 1 : Gain  Gain=0.01*pi/180
  deg/ss to rad/ss : Gain  Gain=pi/180
  deg/ss to rad/ss - 1 : Gain  Gain=pi/180
  dt : Constant  Value=0.01  VectorParams1D=off
  angVelPitch : Outport
  wires:
  Gain1/1 -> Saturation Dynamic/2
  Saturation Dynamic/1 -> Square Root Controller/3(second_ord_lim)
  attitudeErrorPitch/1 -> Product/2, Square Root Controller/1(err)
  Product/1 -> Switch/3
  Square Root Controller/1(correction_rate) -> Switch/1
  Switch/1 -> angVelPitch/1
  ATC.ANG_PIT_P/1 -> Square Root Controller/2(p)
  ATC.ANG_PIT_P - 1/1 -> Product/1
  cdeg/ss to rad/ss - 1/1 -> Switch/2
  ATC.ACCEL_RP_CONTROLLER_MIN_RADSS/1 -> deg/ss to rad/ss - 1/1
  cdeg/ss to rad/ss/1 -> Gain1/1
  ATC.ACCEL_RP_CONTROLLER_MAX_RADSS/1 -> deg/ss to rad/ss/1
  deg/ss to rad/ss/1 -> Saturation Dynamic/1
  deg/ss to rad/ss - 1/1 -> Saturation Dynamic/3
  dt/1 -> Square Root Controller/4(dt)
  Constant/1 -> cdeg/ss to rad/ss/1
  Constant1/1 -> cdeg/ss to rad/ss - 1/1

== system Leader/Ardupilot Attitude Controller/Attitude Controller/input_euler_angle_roll_pitch_euler_rate_yaw()/update_ang_vel_target_from_att_error()/Calc angular velocity target roll ==
  note: Use square root controller if maximum angular acceleration is not zero
  attitudeErrorRoll : Inport
  ATC.ACCEL_RP_CONTROLLER_MAX_RADSS : Constant  Value=720
  ATC.ACCEL_RP_CONTROLLER_MIN_RADSS : Constant  Value=40
  ATC.ACCEL_R_MAX : Constant  Commented=on  Value=108000
  ATC.ACCEL_R_MAX - 1 : Constant  Commented=on  Value=108000
  ATC.ANG_RLL_P : Constant  Value=4.5
  ATC.ANG_RLL_P - 1 : Constant  Value=6.0
  Constant : Constant  Value=0
  Constant1 : Constant  Value=0
  Gain : Gain  Gain=0.5
  Product : Product
  Saturation Dynamic : simulink/Discontinuities/Saturation Dynamic  OutMin=[]  OutMax=[]  OutDataTypeStr=Inherit: Same as second input  OutDataType=fixdt(1, 16)  OutScaling=2^-10  DoSatur=off
  Square Root Controller : MATLAB Function  TreatAsAtomicUnit=on
  Switch : Switch  Criteria=u2 > Threshold  SaturateOnIntegerOverflow=off  InputSameDT=off
  cdeg/ss to rad/ss : Gain  Gain=0.01*pi/180
  cdeg/ss to rad/ss - 1 : Gain  Gain=0.01*pi/180
  deg/ss to rad/ss : Gain  Gain=pi/180
  deg/ss to rad/ss - 1 : Gain  Gain=pi/180
  dt : Constant  Value=0.01  VectorParams1D=off
  angVelRoll : Outport
  wires:
  cdeg/ss to rad/ss - 1/1 -> Switch/2
  ATC.ANG_RLL_P - 1/1 -> Product/1
  ATC.ANG_RLL_P/1 -> Square Root Controller/2(p)
  Switch/1 -> angVelRoll/1
  Square Root Controller/1(correction_rate) -> Switch/1
  dt/1 -> Square Root Controller/4(dt)
  Product/1 -> Switch/3
  attitudeErrorRoll/1 -> Product/2, Square Root Controller/1(err)
  Saturation Dynamic/1 -> Square Root Controller/3(second_ord_lim)
  Gain/1 -> Saturation Dynamic/2
  cdeg/ss to rad/ss/1 -> Gain/1
  ATC.ACCEL_RP_CONTROLLER_MAX_RADSS/1 -> deg/ss to rad/ss/1
  deg/ss to rad/ss/1 -> Saturation Dynamic/1
  ATC.ACCEL_RP_CONTROLLER_MIN_RADSS/1 -> deg/ss to rad/ss - 1/1
  deg/ss to rad/ss - 1/1 -> Saturation Dynamic/3
  Constant1/1 -> cdeg/ss to rad/ss/1
  Constant/1 -> cdeg/ss to rad/ss - 1/1

== system Leader/Ardupilot Attitude Controller/Attitude Controller/input_euler_angle_roll_pitch_euler_rate_yaw()/update_ang_vel_target_from_att_error()/Calc angular velocity target yaw ==
  note: Use square root controller if maximum angular acceleration is not zero
  attitudeErrorYaw : Inport
  ATC.ACCEL_Y_CONTROLLER_MAX_RADSS : Constant  Value=120
  ATC.ACCEL_Y_CONTROLLER_MIN_RADSS : Constant  Value=10
  ATC.ACCEL_Y_MAX : Constant  Commented=on  Value=36000
  ATC.ACCEL_Y_MAX - 1 : Constant  Commented=on  Value=36000
  ATC.ANG_YAW_P : Constant  Value=4.5
  ATC.ANG_YAW_P - 1 : Constant  Value=6.0
  Constant : Constant  Value=0
  Constant1 : Constant  Value=0
  Gain1 : Gain  Gain=0.5
  Product : Product
  Saturation Dynamic : simulink/Discontinuities/Saturation Dynamic  OutMin=[]  OutMax=[]  OutDataTypeStr=Inherit: Same as second input  OutDataType=fixdt(1, 16)  OutScaling=2^-10  DoSatur=off
  Square Root Controller : MATLAB Function  TreatAsAtomicUnit=on
  Switch : Switch  Criteria=u2 > Threshold  SaturateOnIntegerOverflow=off  InputSameDT=off
  cdeg/ss to rad/ss : Gain  Gain=0.01*pi/180
  cdeg/ss to rad/ss - 1 : Gain  Gain=0.01*pi/180
  deg/ss to rad/ss : Gain  Gain=pi/180
  deg/ss to rad/ss - 1 : Gain  Gain=pi/180
  dt : Constant  Value=0.01  VectorParams1D=off
  angVelYaw : Outport
  wires:
  cdeg/ss to rad/ss - 1/1 -> Switch/2
  ATC.ANG_YAW_P - 1/1 -> Product/1
  Switch/1 -> angVelYaw/1
  Square Root Controller/1(correction_rate) -> Switch/1
  Product/1 -> Switch/3
  attitudeErrorYaw/1 -> Product/2, Square Root Controller/1(err)
  Saturation Dynamic/1 -> Square Root Controller/3(second_ord_lim)
  Gain1/1 -> Saturation Dynamic/2
  deg/ss to rad/ss - 1/1 -> Saturation Dynamic/3
  dt/1 -> Square Root Controller/4(dt)
  ATC.ACCEL_Y_CONTROLLER_MAX_RADSS/1 -> deg/ss to rad/ss/1
  cdeg/ss to rad/ss/1 -> Gain1/1
  deg/ss to rad/ss/1 -> Saturation Dynamic/1
  ATC.ACCEL_Y_CONTROLLER_MIN_RADSS/1 -> deg/ss to rad/ss - 1/1
  ATC.ANG_YAW_P/1 -> Square Root Controller/2(p)
  Constant/1 -> cdeg/ss to rad/ss/1
  Constant1/1 -> cdeg/ss to rad/ss - 1/1

== system Leader/Ardupilot Attitude Controller/Attitude Controller/input_euler_angle_roll_pitch_euler_rate_yaw()/Feedforward enabled/input shaping/input shaping pitch angle ==
  note: AC_AttitudeControl::input_shaping_angle(float error_angle, float input_tc, float accel_max, float target_ang_vel, float desired_ang_vel, float max_ang_vel, float dt)
      | Calculation of velocity correction from an angle error. The angular velocity has acceleration and deceleration limits including basic jerk limiting using _input_tc.
      |
      | Function is called from input_shaping_angle(float error_angle, float smoothing_gain, float accel_max, float target_ang_vel, float dt) as input_shaping_angle(error_angle, smoothing_gain, accel_max, target_ang_vel, 0.0f, 0.0f, dt), so desired_ang_vel = 0 and max_ang_vel = 0
  pitchAngleErr : Inport
  pitchRateTarIn : Inport  Port=2
  pitchAccelMax : Inport  Port=3
  ATC.INPUT_TC : Constant  Value=0.15  VectorParams1D=off
  Constant3 : Constant  Value=0  VectorParams1D=off
  MATLAB Function : MATLAB Function  TreatAsAtomicUnit=on
  MATLAB Function1 : MATLAB Function  TreatAsAtomicUnit=on
  Square Root Controller : MATLAB Function  TreatAsAtomicUnit=on
  Square Root Controller1 : Subsystem  Commented=on  TreatAsAtomicUnit=on
  calc p from input_tc : Subsystem
  dt : Constant  Value=0.01  VectorParams1D=off
  eulerPitchRateTar : Outport
  wires:
  MATLAB Function1/1(eulerRateTar) -> eulerPitchRateTar/1
  [accelMax] -> Square Root Controller/3(second_ord_lim)
  Square Root Controller/1(correction_rate) -> MATLAB Function1/1(desiredAngVel)
  calc p from input_tc/1(p) -> Square Root Controller/2(p)
  ATC.INPUT_TC/1 -> calc p from input_tc/1(input_tc)
  pitchAccelMax/1 -> [accelMax]
  MATLAB Function/1(radLim) -> Square Root Controller/1(err)
  pitchAngleErr/1 -> MATLAB Function/1(radIn)
  pitchRateTarIn/1 -> MATLAB Function1/2(targetAngVel)
  dt/1 -> MATLAB Function1/4(dt), Square Root Controller/4(dt)
  Constant3/1 -> MATLAB Function1/5(input_tc)
  [accelMax] -> MATLAB Function1/3(accelMax)

== system Leader/Ardupilot Attitude Controller/Attitude Controller/input_euler_angle_roll_pitch_euler_rate_yaw()/Feedforward enabled/input shaping/input shaping roll angle ==
  note: AC_AttitudeControl::input_shaping_angle(float error_angle, float input_tc, float accel_max, float target_ang_vel, float desired_ang_vel, float max_ang_vel, float dt)
      | Calculation of velocity correction from an angle error. The angular velocity has acceleration and deceleration limits including basic jerk limiting using _input_tc.
      |
      | Function is called from input_shaping_angle(float error_angle, float smoothing_gain, float accel_max, float target_ang_vel, float dt) as input_shaping_angle(error_angle, smoothing_gain, accel_max, target_ang_vel, 0.0f, 0.0f, dt), so desired_ang_vel = 0 and max_ang_vel = 0
  rollAngleErr : Inport
  rollRateTarIn : Inport  Port=2
  rollAccelMax : Inport  Port=3
  ATC.INPUT_TC : Constant  Value=0.15  VectorParams1D=off
  Constant3 : Constant  Value=0  VectorParams1D=off
  MATLAB Function : MATLAB Function  TreatAsAtomicUnit=on
  MATLAB Function1 : MATLAB Function  TreatAsAtomicUnit=on
  Square Root Controller : MATLAB Function  TreatAsAtomicUnit=on
  Square Root Controller1 : Subsystem  Commented=on  TreatAsAtomicUnit=on
  calc p from input_tc : Subsystem
  dt : Constant  Value=0.01  VectorParams1D=off
  eulerRollRateTar : Outport
  wires:
  rollAngleErr/1 -> MATLAB Function/1(radIn)
  MATLAB Function/1(radLim) -> Square Root Controller/1(err)
  rollAccelMax/1 -> [accelMax]
  ATC.INPUT_TC/1 -> calc p from input_tc/1(input_tc)
  calc p from input_tc/1(p) -> Square Root Controller/2(p)
  Square Root Controller/1(correction_rate) -> MATLAB Function1/1(desiredAngVel)
  [accelMax] -> Square Root Controller/3(second_ord_lim)
  [accelMax] -> MATLAB Function1/3(accelMax)
  MATLAB Function1/1(eulerRateTar) -> eulerRollRateTar/1
  rollRateTarIn/1 -> MATLAB Function1/2(targetAngVel)
  dt/1 -> MATLAB Function1/4(dt), Square Root Controller/4(dt)
  Constant3/1 -> MATLAB Function1/5(input_tc)

== system Leader/Ardupilot Attitude Controller/Attitude Controller/input_euler_angle_roll_pitch_euler_rate_yaw()/Feedforward enabled/input shaping/input shaping yaw rate ==
  note: AC_AttitudeControl::input_shaping_ang_vel()
      | Limits the maximum acceleration resulting from the target yaw rate, so that the target yaw rate is slewed towards the input rate
  yawRateDes : Inport
  yawRateTar : Inport  Port=2
  eulerAccelMax : Inport  Port=3
  MATLAB Function1 : MATLAB Function
  PILOT_Y_RATE_TC : Constant  Value=0.15  VectorParams1D=off
  Square Root Controller : Subsystem  Commented=on  TreatAsAtomicUnit=on
  dt : Constant  Value=0.01  VectorParams1D=off
  eulerYawRateTar : Outport
  wires:
  yawRateDes/1 -> MATLAB Function1/1(desiredAngVel)
  eulerAccelMax/1 -> MATLAB Function1/3(accelMax)
  MATLAB Function1/1(eulerRateTar) -> eulerYawRateTar/1
  yawRateTar/1 -> MATLAB Function1/2(targetAngVel)
  dt/1 -> MATLAB Function1/4(dt)
  PILOT_Y_RATE_TC/1 -> MATLAB Function1/5(input_tc)

== system Leader/Ardupilot Attitude Controller/Attitude Controller/input_euler_angle_roll_pitch_euler_rate_yaw()/thrust_heading_rotation_angles()/Yaw error limitation/Yaw limiting and recalculation of attitudeTarget ==
  note: Limit yaw error and calculate new attitudeTarget and attitudeError
  note: Create new attitudeError with limited yaw error
  note: Calculate new attitudeTarget with limited yawVecCorrection
  note: Limit yaw error based on maximum acceleration
  attitudeErrorIn : Inport
  thrustVecCorrection : Inport  Port=2
  attitudeBody : Inport  Port=3
  Enable : EnablePort
  ATC.ACCEL_Y_CONTROLLER_MAX_RADSS : Constant  Value=2.0944
  ATC.ANG_YAW_P : Constant  Value=8.0
  Constant2 : Constant  Value=0
  Demux : Demux  Outputs=2
  Divide : Product  Inputs=*/
  Gain : Gain  Gain=-1
  MATLAB Function : MATLAB Function  TreatAsAtomicUnit=on
  MATLAB Function1 : MATLAB Function  TreatAsAtomicUnit=on
  MATLAB Function5 : MATLAB Function  TreatAsAtomicUnit=on
  MATLAB Function9 : MATLAB Function  TreatAsAtomicUnit=on
  MinMax : MinMax  Inputs=2
  MinMax1 : MinMax  Function=max  Inputs=2
  Mux : Mux  Inputs=3
  Mux1 : Mux  Inputs=3
  Selector : Selector  InputPortWidth=3  IndexOptions=Index vector (dialog)  Indices=[3]  OutputSizes=1
  Selector1 : Selector  InputPortWidth=3  IndexOptions=Index vector (dialog)  Indices=[1 2]  OutputSizes=1
  attitudeTarget : Outport
  attitudeError : Outport  Port=2
  wires:
  ATC.ACCEL_Y_CONTROLLER_MAX_RADSS/1 -> Divide/1
  ATC.ANG_YAW_P/1 -> Divide/2
  [attitudeError] -> Selector/1
  Selector/1 -> MinMax/1
  Divide/1 -> MinMax/2, Gain/1
  MinMax/1 -> MinMax1/1
  Gain/1 -> MinMax1/2
  MinMax1/1 -> MATLAB Function/1(radIn)
  MATLAB Function/1(radLim) -> Mux1/3, Mux/3
  Constant2/1 -> Mux/2, Mux/1
  Mux/1 -> MATLAB Function5/1(vec)
  MATLAB Function5/1(q) -> MATLAB Function9/2(q2)  "yawVecCorrection"
  MATLAB Function9/1(qRes) -> MATLAB Function1/2(q2)
  thrustVecCorrection/1 -> MATLAB Function9/1(q1)
  attitudeBody/1 -> MATLAB Function1/1(q1)
  MATLAB Function1/1(qRes) -> attitudeTarget/1
  Mux1/1 -> attitudeError/1
  attitudeErrorIn/1 -> [attitudeError]
  [attitudeError] -> Selector1/1
  Selector1/1 -> Demux/1
  Demux/1 -> Mux1/1
  Demux/2 -> Mux1/2

== system Leader/Ardupilot Attitude Controller/Attitude Controller/input_euler_angle_roll_pitch_euler_rate_yaw()/Feedforward enabled/input shaping/input shaping pitch angle/Square Root Controller1 ==
  sqrt_controller : TriggerPort  TriggerType=function-call  IsSimulinkFunction=on  FunctionName=sqrt_controller  FunctionVisibility=scoped  VariantControl=(inherit)
  Square Root Controller : MATLAB Function  TreatAsAtomicUnit=on
  err : ArgIn  DisableCoverage=on  OutDataTypeStr=single  ArgumentName=err
  p : ArgIn  DisableCoverage=on  Port=2  OutDataTypeStr=single  ArgumentName=p
  second_ord_lim : ArgIn  DisableCoverage=on  Port=3  OutDataTypeStr=single  ArgumentName=second_ord_lim
  dt : ArgIn  DisableCoverage=on  Port=4  OutDataTypeStr=single  ArgumentName=dt
  correctionRate : ArgOut  DisableCoverage=on  OutDataTypeStr=single  ArgumentName=correctionRate
  wires:
  err/1 -> Square Root Controller/1(err)
  p/1 -> Square Root Controller/2(p)
  second_ord_lim/1 -> Square Root Controller/3(second_ord_lim)
  Square Root Controller/1(correction_rate) -> correctionRate/1
  dt/1 -> Square Root Controller/4(dt)

== system Leader/Ardupilot Attitude Controller/Attitude Controller/input_euler_angle_roll_pitch_euler_rate_yaw()/Feedforward enabled/input shaping/input shaping pitch angle/calc p from input_tc ==
  note: Calculation of proportional factor of square root controller.
      | Based on function argument of sqrt_controller() in AC_AttitudeControl::input_shaping_angle()
  input_tc : Inport
  Constant2 : Constant  Value=0.01  OutDataTypeStr=double
  Constant3 : Constant  OutDataTypeStr=single
  Divide : Product  Inputs=*/
  Max : MinMax  Function=max  Inputs=2
  p : Outport
  wires:
  Constant2/1 -> Max/2
  Max/1 -> Divide/2
  Constant3/1 -> Divide/1
  input_tc/1 -> Max/1
  Divide/1 -> p/1

== system Leader/Ardupilot Attitude Controller/Attitude Controller/input_euler_angle_roll_pitch_euler_rate_yaw()/Feedforward enabled/input shaping/input shaping roll angle/Square Root Controller1 ==
  sqrt_controller : TriggerPort  TriggerType=function-call  IsSimulinkFunction=on  FunctionName=sqrt_controller  FunctionVisibility=scoped  VariantControl=(inherit)  SampleTimeType=periodic  SampleTime=-1
  Square Root Controller : MATLAB Function  TreatAsAtomicUnit=on
  err : ArgIn  DisableCoverage=on  OutDataTypeStr=single  ArgumentName=err
  p : ArgIn  DisableCoverage=on  Port=2  OutDataTypeStr=single  ArgumentName=p
  second_ord_lim : ArgIn  DisableCoverage=on  Port=3  OutDataTypeStr=single  ArgumentName=second_ord_lim
  dt : ArgIn  DisableCoverage=on  Port=4  OutDataTypeStr=single  ArgumentName=dt
  correctionRate : ArgOut  DisableCoverage=on  OutDataTypeStr=single  ArgumentName=correctionRate
  wires:
  err/1 -> Square Root Controller/1(err)
  p/1 -> Square Root Controller/2(p)
  second_ord_lim/1 -> Square Root Controller/3(second_ord_lim)
  Square Root Controller/1(correction_rate) -> correctionRate/1
  dt/1 -> Square Root Controller/4(dt)

== system Leader/Ardupilot Attitude Controller/Attitude Controller/input_euler_angle_roll_pitch_euler_rate_yaw()/Feedforward enabled/input shaping/input shaping roll angle/calc p from input_tc ==
  note: Calculation of proportional factor of square root controller.
      | Based on function argument of sqrt_controller() in AC_AttitudeControl::input_shaping_angle()
  input_tc : Inport
  Constant2 : Constant  Value=0.01  OutDataTypeStr=double
  Constant3 : Constant  OutDataTypeStr=single
  Divide : Product  Inputs=*/
  Max : MinMax  Function=max  Inputs=2
  p : Outport
  wires:
  Constant2/1 -> Max/2
  Max/1 -> Divide/2
  Constant3/1 -> Divide/1
  input_tc/1 -> Max/1
  Divide/1 -> p/1

== system Leader/Ardupilot Attitude Controller/Attitude Controller/input_euler_angle_roll_pitch_euler_rate_yaw()/Feedforward enabled/input shaping/input shaping yaw rate/Square Root Controller ==
  sqrt_controller : TriggerPort  TriggerType=function-call  IsSimulinkFunction=on  FunctionName=sqrt_controller  FunctionVisibility=scoped  VariantControl=(inherit)
  Square Root Controller : MATLAB Function  TreatAsAtomicUnit=on
  output : ArgIn  DisableCoverage=on  OutDataTypeStr=single  ArgumentName=err
  p : ArgIn  DisableCoverage=on  Port=2  OutDataTypeStr=single  ArgumentName=p
  D_max : ArgIn  DisableCoverage=on  Port=3  OutDataTypeStr=single  ArgumentName=second_ord_lim
  output1 : ArgIn  DisableCoverage=on  Port=4  OutDataTypeStr=single  ArgumentName=dt
  correctionRate : ArgOut  DisableCoverage=on  OutDataTypeStr=single  ArgumentName=correctionRate
  wires:
  output/1 -> Square Root Controller/1(err)
  p/1 -> Square Root Controller/2(p)
  D_max/1 -> Square Root Controller/3(second_ord_lim)
  Square Root Controller/1(correction_rate) -> correctionRate/1
  output1/1 -> Square Root Controller/4(dt)

== matlab function Leader/SMC Position Controller/MATLAB Function4 ==
  data: Sz_prev input; zintg output; curr_err input; prev_err input; zintg_prev input
function zintg = trap_intg(Sz_prev, curr_err, prev_err, zintg_prev)

% Define timestep size and boundary layer thicknesses
Ts = 0.02;
Bz = 0.3;
zintg = zintg_prev;

if(abs(Sz_prev) < Bz)
    zintg = zintg_prev + (curr_err + prev_err) * (Ts/2);
end

== matlab function Leader/Ardupilot Attitude Controller/Rate Controller/PID Roll Rate/I/Integrator ==
  data: error input; integrator_out output; integrator input; limit_flg input; ki input; i_max input; dt input
function integrator_out = fcn(error, integrator, limit_flg, ki, i_max, dt)
% Code is based on AC_PID::update_i() in AC_PID.cpp.

% Check plausibility of input parameters
if (ki ~= 0 && dt > 0)
    % Only allow integration if limit is not set or the absolute sum of the
    % integrator would be reduced.
    if (~limit_flg || (integrator > 0 && error < 0) || (integrator < 0 && error > 0))
        integrator_out = integrator + error * ki * dt;
        integrator_out = max( min(integrator_out, i_max), -i_max);
    else % Otherwise, keep old integrator value
        integrator_out = integrator;
    end
else % Reset integrator if input parameters are not plausible
    integrator_out = 0.0;
end
